simulink model "soc_luenbege"  (R2023b)
settings: Solver=VariableStepAuto  StartTime=0.0  StopTime=10.0  RelTol=1e-3
settings Model: Creator=CSC  LastModifiedBy=CSC

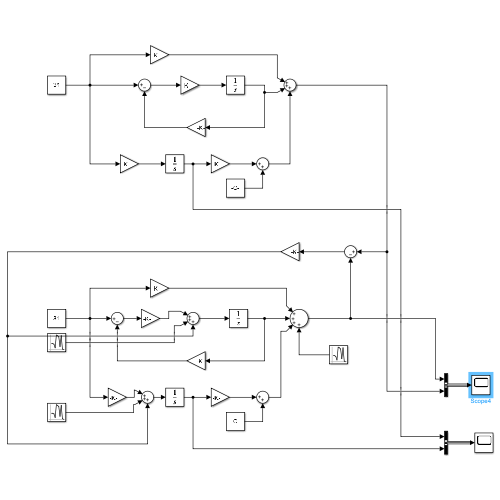
[thumbnail: Simulink's stored preview of the top-level diagram]
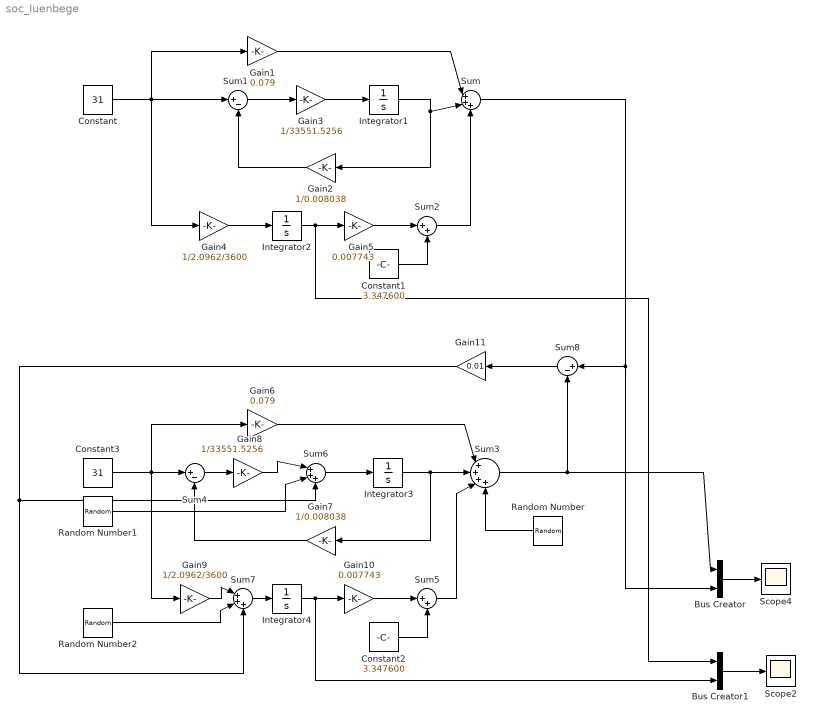
== system soc_luenbege ==
  Bus Creator : BusCreator  Inputs=2
  Bus Creator1 : BusCreator  Inputs=2
  Constant : Constant  Value=31
  Constant1 : Constant  Value=3.347600
  Constant2 : Constant  Value=3.347600
  Constant3 : Constant  Value=31
  Gain1 : Gain  Gain=0.079
  Gain10 : Gain  Gain=0.007743
  Gain11 : Gain  Gain=0.01
  Gain2 : Gain  Gain=1/0.008038
  Gain3 : Gain  Gain=1/33551.5256
  Gain4 : Gain  Gain=1/2.0962/3600
  Gain5 : Gain  Gain=0.007743
  Gain6 : Gain  Gain=0.079
  Gain7 : Gain  Gain=1/0.008038
  Gain8 : Gain  Gain=1/33551.5256
  Gain9 : Gain  Gain=1/2.0962/3600
  Integrator{1..4} (4 alike) : Integrator
  Random Number : RandomNumber  Variance=0.0001  SampleTime=0.1
  Random Number1 : RandomNumber  Variance=0.0001  SampleTime=0.1
  Random Number2 : RandomNumber  Variance=0.0001  SampleTime=0.1
  Scope2 : Scope
  Scope4 : Scope
  Sum : Sum  Inputs=|+++
  Sum1 : Sum  Inputs=|+-
  Sum2 : Sum  Inputs=|++
  Sum3 : Sum  Inputs=|++++
  Sum4 : Sum  Inputs=|+-
  Sum5 : Sum  Inputs=|++
  Sum6 : Sum  Inputs=|+++
  Sum7 : Sum  Inputs=|+++
  Sum8 : Sum  Inputs=|+-
  wires:
  Sum/1 -> Bus Creator/2, Sum8/1
  Constant/1 -> Gain4/1, Gain1/1, Sum1/1
  Gain1/1 -> Sum/1
  Integrator1/1 -> Gain2/1, Sum/2
  Gain2/1 -> Sum1/2
  Sum1/1 -> Gain3/1
  Gain3/1 -> Integrator1/1
  Gain4/1 -> Integrator2/1
  Sum2/1 -> Sum/3
  Integrator2/1 -> Bus Creator1/1, Gain5/1
  Gain5/1 -> Sum2/1
  Constant1/1 -> Sum2/2
  Sum3/1 -> Bus Creator/1, Sum8/2
  Constant3/1 -> Gain9/1, Gain6/1, Sum4/1
  Gain6/1 -> Sum3/1
  Gain10/1 -> Sum5/1
  Sum4/1 -> Gain8/1
  Constant2/1 -> Sum5/2
  Sum5/1 -> Sum3/3
  Integrator4/1 -> Bus Creator1/2, Gain10/1
  Integrator3/1 -> Gain7/1, Sum3/2
  Gain7/1 -> Sum4/2
  Random Number/1 -> Sum3/4
  Gain8/1 -> Sum6/1
  Sum6/1 -> Integrator3/1
  Random Number1/1 -> Sum6/2
  Gain9/1 -> Sum7/1
  Sum7/1 -> Integrator4/1
  Random Number2/1 -> Sum7/2
  Sum8/1 -> Gain11/1
  Gain11/1 -> Sum6/3, Sum7/3
  Bus Creator/1 -> Scope4/1
  Bus Creator1/1 -> Scope2/1
